simulink model "Acc_and_Gyro_Handling"  (R2018a)
settings: Solver=VariableStepAuto  StartTime=0.0  StopTime=30  RelTol=1e-3
undefined symbols (not defined in the file): DiscIntNeverNeededParam, GyroSet
libraries: simulink x4
settings Model: Creator=Hannes  LastModifiedBy=Hannes

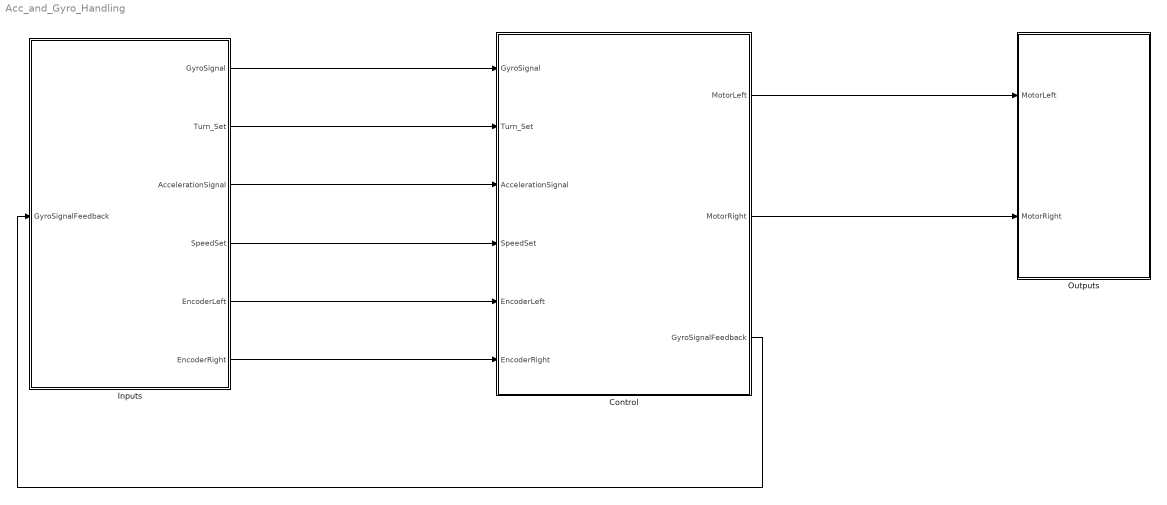
== system Acc_and_Gyro_Handling ==
  Control : Subsystem
  Inputs : Subsystem
  "Outputs " : Subsystem
  wires:
  Inputs/1(GyroSignal) -> Control/1(GyroSignal)
  Inputs/2(Turn_Set) -> Control/2(Turn_Set)
  Inputs/3(AccelerationSignal) -> Control/3(AccelerationSignal)
  Inputs/4(SpeedSet) -> Control/4(SpeedSet)
  Inputs/5(EncoderLeft) -> Control/5(EncoderLeft)
  Inputs/6(EncoderRight) -> Control/6(EncoderRight)
  Control/1(MotorLeft) -> "Outputs "/1(MotorLeft)
  Control/2(MotorRight) -> "Outputs "/2(MotorRight)
  Control/3(GyroSignalFeedback) -> Inputs/1("GyroSignalFeedback ")

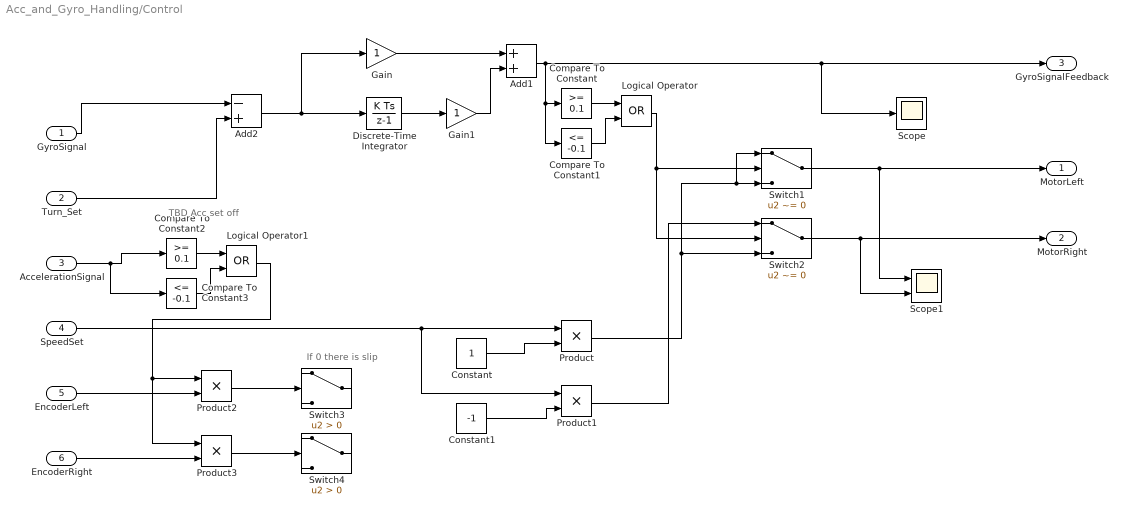
== system Acc_and_Gyro_Handling/Control ==
  note: If 0 there is slip
  note: TBD Acc set off
  GyroSignal : Inport
  Turn_Set : Inport  Port=2
  AccelerationSignal : Inport  Port=3
  SpeedSet : Inport  Port=4
  EncoderLeft : Inport  Port=5
  EncoderRight : Inport  Port=6
  Add1 : Sum
  Add2 : Sum  Inputs=-+
  Compare To Constant : simulink/Logic and Bit Operations/Compare To Constant  relop=>=  const=0.1  OutDataTypeStr=boolean
  Compare To Constant1 : simulink/Logic and Bit Operations/Compare To Constant  relop=<=  const=-0.1  OutDataTypeStr=boolean
  Compare To Constant2 : simulink/Logic and Bit Operations/Compare To Constant  relop=>=  const=0.1  OutDataTypeStr=boolean
  Compare To Constant3 : simulink/Logic and Bit Operations/Compare To Constant  relop=<=  const=-0.1  OutDataTypeStr=boolean
  Constant : Constant
  Constant1 : Constant  Value=-1
  Discrete-Time Integrator : DiscreteIntegrator  SampleTime=-1  ICPrevOutput=DiscIntNeverNeededParam  ICPrevScaledInput=DiscIntNeverNeededParam
  Gain : Gain
  Gain1 : Gain
  Logical Operator : Logic  Operator=OR  AllPortsSameDT=off  OutDataTypeStr=boolean
  Logical Operator1 : Logic  Operator=OR  AllPortsSameDT=off  OutDataTypeStr=boolean
  Product{,1..3} (4 alike) : Product
  Scope : Scope
  Scope1 : Scope  NumInputPorts=2
  Switch1 : Switch  Criteria=u2 ~= 0  Threshold=GyroSet
  Switch2 : Switch  Criteria=u2 ~= 0  Threshold=GyroSet
  Switch3 : Switch  Criteria=u2 > Threshold
  Switch4 : Switch  Criteria=u2 > Threshold
  MotorLeft : Outport
  MotorRight : Outport  Port=2
  GyroSignalFeedback : Outport  Port=3
  wires:
  Gain1/1 -> Add1/2
  Discrete-Time Integrator/1 -> Gain1/1
  Gain/1 -> Add1/1
  Add2/1 -> Gain/1, Discrete-Time Integrator/1
  GyroSignal/1 -> Add2/1
  Turn_Set/1 -> Add2/2
  Add1/1 -> Scope/1, GyroSignalFeedback/1, Compare To Constant/1, Compare To Constant1/1
  SpeedSet/1 -> Product1/1, Product/1
  Constant/1 -> Product/2
  Product/1 -> Switch2/3, Switch1/3, Switch1/1
  Switch2/1 -> Scope1/2, MotorRight/1
  Switch1/1 -> Scope1/1, MotorLeft/1
  Constant1/1 -> Product1/2
  Product1/1 -> Switch2/1
  Compare To Constant/1 -> Logical Operator/1
  Compare To Constant1/1 -> Logical Operator/2
  Logical Operator/1 -> Switch2/2, Switch1/2
  EncoderLeft/1 -> Product2/2
  EncoderRight/1 -> Product3/2
  Compare To Constant2/1 -> Logical Operator1/1
  Compare To Constant3/1 -> Logical Operator1/2
  AccelerationSignal/1 -> Compare To Constant3/1, Compare To Constant2/1
  Logical Operator1/1 -> Product3/1, Product2/1
  Product2/1 -> Switch3/2
  Product3/1 -> Switch4/2

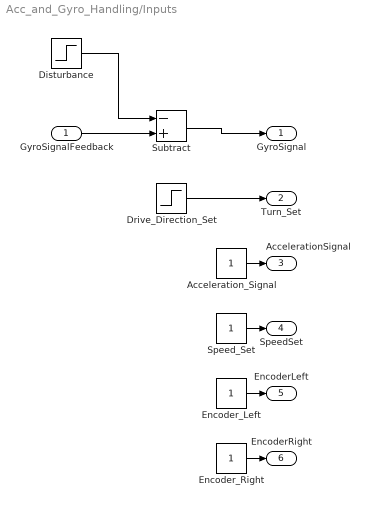
== system Acc_and_Gyro_Handling/Inputs ==
  "GyroSignalFeedback " : Inport
  Acceleration_Signal : Constant
  Disturbance : Step  Time=8  Before=-4  After=0  SampleTime=0
  Drive_Direction_Set : Step  Time=5  Before=3  After=0  SampleTime=0
  Encoder_Left : Constant
  Encoder_Right : Constant
  Speed_Set : Constant
  Subtract : Sum  Inputs=-+
  GyroSignal : Outport
  Turn_Set : Outport  Port=2
  AccelerationSignal : Outport  Port=3
  SpeedSet : Outport  Port=4
  EncoderLeft : Outport  Port=5
  EncoderRight : Outport  Port=6
  wires:
  "GyroSignalFeedback "/1 -> Subtract/2
  Speed_Set/1 -> SpeedSet/1
  Drive_Direction_Set/1 -> Turn_Set/1
  Encoder_Left/1 -> EncoderLeft/1
  Acceleration_Signal/1 -> AccelerationSignal/1
  Encoder_Right/1 -> EncoderRight/1
  Subtract/1 -> GyroSignal/1
  Disturbance/1 -> Subtract/1

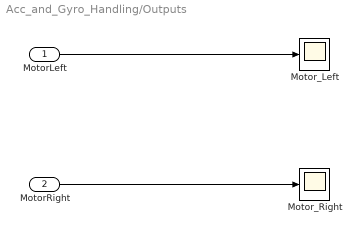
== system Acc_and_Gyro_Handling/Outputs  ==
  MotorLeft : Inport
  MotorRight : Inport  Port=2
  Motor_Left : Scope
  Motor_Right : Scope
  wires:
  MotorLeft/1 -> Motor_Left/1
  MotorRight/1 -> Motor_Right/1
